simulink subsystem "model_inductance"  (R2024a)
settings: Solver=VariableStepAuto  StartTime=0.0  StopTime=10.0  RelTol=1e-3
values from neighbouring files (symbols this model uses):
  a = 1 / 0.0058231    (= 171.729834624)    [maglev_parameters.m]
  L0 = 0.5*1e-3    (= 0.0005)    [maglev_parameters.m]
  Ld = 0.017521    [maglev_parameters.m]
settings Model: Creator=Bocchio  LastModifiedBy=Bocchio

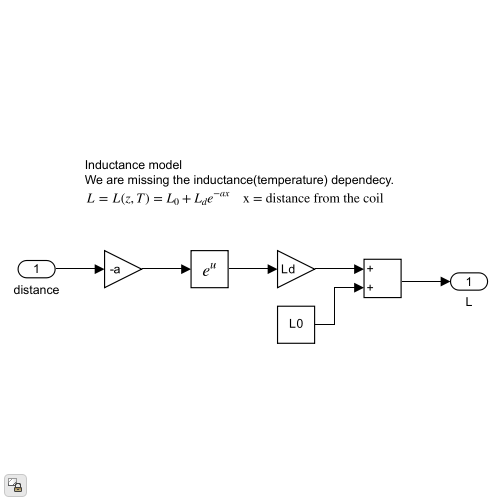
[thumbnail: Simulink's stored preview of the top-level diagram]
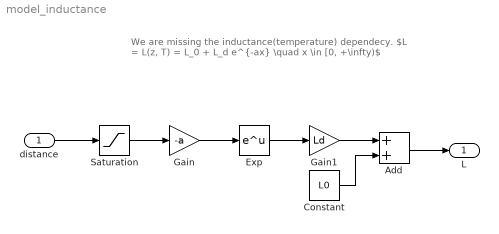
== system model_inductance ==
  note: We are missing the inductance(temperature) dependecy.
      | $L = L(z, T) = L_0 + L_d e^{-ax} \quad x \in [0, +\infty)$
  distance : Inport
  Add : Sum
  Constant : Constant  Value=L0
  Exp : Math
  Gain : Gain  Gain=-a
  Gain1 : Gain  Gain=Ld
  Saturation : Saturate  UpperLimit=+inf  LowerLimit=0
  L : Outport
  wires:
  distance/1 -> Saturation/1
  Add/1 -> L/1
  Constant/1 -> Add/2
  Gain1/1 -> Add/1
  Exp/1 -> Gain1/1
  Gain/1 -> Exp/1
  Saturation/1 -> Gain/1
